simulink model "VVI_REPLACEMENT"  (R2022b)
settings: Solver=FixedStepAuto  StartTime=0.0  StopTime=100  FixedStep=1e-3  RelTol=1e-3  EnableMultiTasking=on
undefined symbols (not defined in the file): D1, D10, D12, D13, D2, D3, D5, D9, PTA1, PTA2, PTB9, PTC17, PTC4, PTD0, PTD1, PTD3
libraries: frdmk64flib x8
settings Model: ExtModeTrigDuration=5  Creator=aldenluscher  LastModifiedBy=aldenluscher
settings OptimizationCC: EnhancedBackFolding=on  PassReuseOutputArgsAs=Individual arguments  ZeroExternalMemoryAtStartup=off  ZeroInternalMemoryAtStartup=off  MaxStackSize=64  OptimizeBlockOrder=speed  DifferentSizesBufferReuse=on  OptimizationCustomize=off  EfficientTunableParamExpr=on
settings DebuggingCC: ParameterTunabilityLossMsg=error
settings HardwareCC: ProdBitPerPointer=32  ProdBitPerSizeT=32  ProdBitPerPtrDiffT=32  ProdLargestAtomicInteger=Long  ProdLargestAtomicFloat=Double  ProdWordSize=32  ProdHWDeviceType=ARM Compatible->ARM Cortex
settings SFSimCC: MATLABDynamicMemAlloc=off
settings RTWCC: Description=Embedded Coder  SystemTargetFile=ert.tlc  HardwareBoard=NXP FRDM-K64F  TLCOptions="-aInlineSetEventsForThisBaseRateFcn=TLC_FALSE -aSuppressMultiTaskScheduler=TLC_FALSE  -aRateBasedStepFcn=0"  TemplateMakefile=ert_default_tmf  Toolchain=GNU Tools for ARM Embedded Processors
settings CodeAppCC: ForceParamTrailComments=on  IgnoreCustomStorageClasses=off  OperatorAnnotations=on  SimulinkDataObjDesc=on  SFDataObjDesc=on  InsertBlockDesc=on
settings ERTTargetCC: ExtModeTransport=4  ExtModeMexFile=sendToCommService

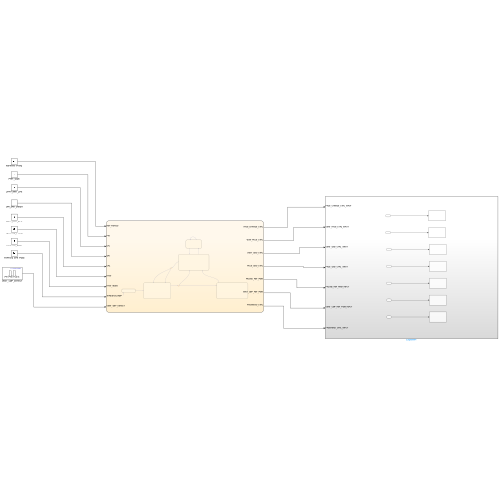
[thumbnail: Simulink's stored preview of the top-level diagram]
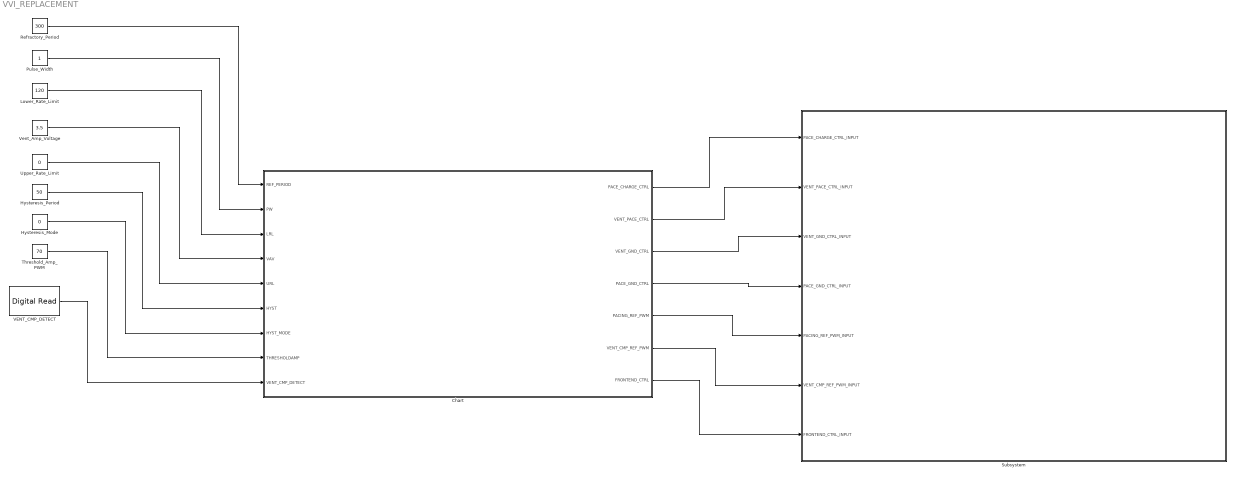
== system VVI_REPLACEMENT ==
  Chart : Stateflow chart  TreatAsAtomicUnit=on
      settings: PortSchema="{\"entries\":[{\"content\":{\"sides\":[{\"content\":{\"connectorIds\":[\"In1\",\"In2\",\"In3\",\"In4\",\"In5\",\"In7\",\"In6\",\"In9\",\"In8\"]},\"type\":\"ConnectorPlacement.EquallySpacedRectSide\",\"uuid\":\"2ae54867-0d42-4dc9-a711-c3558df1a1e5\"},{\"content\":{\"connectorIds\":[\"Out1\",\"Out2\",\"Out3\",\"Out4\",\"Out5\",\"Out6\",\"Out7\"],\"side\":\"RIGHT\"},\"type\":\"ConnectorPlacement.EquallySpacedRectSide\",\"uuid\":\"0827b622-949a-4894-bfc3-fcfa9f1c5c6f\"},{\"content\":{\"connectorIds\":[],\"side\":\"TOP\"},\"type\":\"ConnectorPlacement.EquallySpacedRectSide\",\"uuid\":\"b2dc8d34-414d-4327-a079-fe4380aaf0f4\"}]},\"type\":\"ConnectorPlacement.EquallySpacedConnector\",\"uuid\":\"8b20b6f2-40a5-4126-b6c0-e8236ebafa56\"}],\"packageUris\":[\"http://schema.mathworks.com/mf0/Connector/R2020b\"],\"version\":\"1.0\"}"
  Hysteresis_Mode : Constant  Value=0
  Hysteresis_Period : Constant  Value=50
  Lower_Rate_Limit : Constant  Value=120
  Pulse_Width : Constant
  Refractory_Period : Constant  Value=300
  Subsystem : Subsystem
  Threshold_Amp_PWM : Constant  Value=70
  Upper_Rate_Limit : Constant  Value=0
  VENT_CMP_DETECT : frdmk64flib/Digital Read  Whichpin=PTC17 (D1)  SampleTime=-1
  Vent_Amp_Voltage : Constant  Value=3.5
  wires:
  VENT_CMP_DETECT/1 -> Chart/8(VENT_CMP_DETECT)
  Threshold_Amp_PWM/1 -> Chart/9(THRESHOLDAMP)
  Chart/3(VENT_GND_CTRL) -> Subsystem/3(VENT_GND_CTRL_INPUT)
  Refractory_Period/1 -> Chart/1(REF_PERIOD)
  Vent_Amp_Voltage/1 -> Chart/4(VAV)
  Upper_Rate_Limit/1 -> Chart/5(URL)
  Chart/5(PACING_REF_PWM) -> Subsystem/5(PACING_REF_PWM_INPUT)
  Chart/6(VENT_CMP_REF_PWM) -> Subsystem/6(VENT_CMP_REF_PWM_INPUT)
  Hysteresis_Period/1 -> Chart/7(HYST)
  Hysteresis_Mode/1 -> Chart/6(HYST_MODE)
  Chart/2(VENT_PACE_CTRL) -> Subsystem/2(VENT_PACE_CTRL_INPUT)
  Chart/1(PACE_CHARGE_CTRL) -> Subsystem/1(PACE_CHARGE_CTRL_INPUT)
  Lower_Rate_Limit/1 -> Chart/3(LRL)
  Chart/7(FRONTEND_CTRL) -> Subsystem/7(FRONTEND_CTRL_INPUT)
  Pulse_Width/1 -> Chart/2(PW)
  Chart/4(PACE_GND_CTRL) -> Subsystem/4(PACE_GND_CTRL_INPUT)

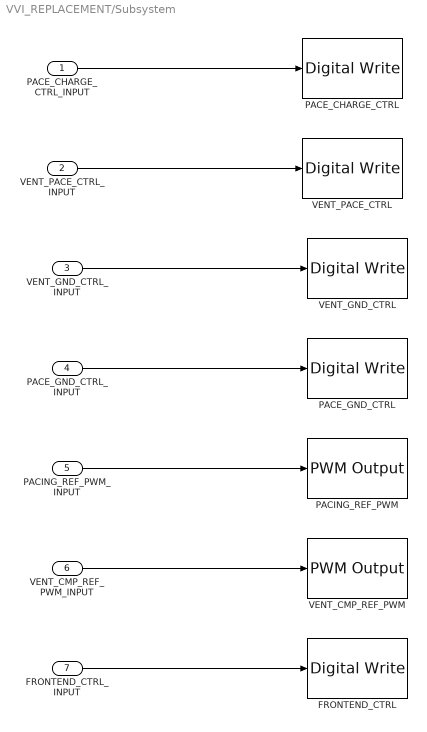
== system VVI_REPLACEMENT/Subsystem ==
  PACE_CHARGE_CTRL_INPUT : Inport
  VENT_PACE_CTRL_INPUT : Inport  Port=2
  VENT_GND_CTRL_INPUT : Inport  Port=3
  PACE_GND_CTRL_INPUT : Inport  Port=4
  PACING_REF_PWM_INPUT : Inport  Port=5
  VENT_CMP_REF_PWM_INPUT : Inport  Port=6
  FRONTEND_CTRL_INPUT : Inport  Port=7
  FRONTEND_CTRL : frdmk64flib/Digital Write  Whichpin=PTD1 (D13)
  PACE_CHARGE_CTRL : frdmk64flib/Digital Write  Whichpin=PTB9 (D2)
  PACE_GND_CTRL : frdmk64flib/Digital Write  Whichpin=PTD0 (D10)
  PACING_REF_PWM : frdmk64flib/PWM Output  Whichpin=PTA2 (D5)  InitialFrequency=2000  InitialDutyCycle=0
  VENT_CMP_REF_PWM : frdmk64flib/PWM Output  Whichpin=PTA1 (D3)  InitialFrequency=2000  InitialDutyCycle=0
  VENT_GND_CTRL : frdmk64flib/Digital Write  Whichpin=PTD3 (D12)
  VENT_PACE_CTRL : frdmk64flib/Digital Write  Whichpin=PTC4 (D9)
  wires:
  VENT_PACE_CTRL_INPUT/1 -> VENT_PACE_CTRL/1
  PACE_GND_CTRL_INPUT/1 -> PACE_GND_CTRL/1
  PACE_CHARGE_CTRL_INPUT/1 -> PACE_CHARGE_CTRL/1
  PACING_REF_PWM_INPUT/1 -> PACING_REF_PWM/1
  VENT_GND_CTRL_INPUT/1 -> VENT_GND_CTRL/1
  VENT_CMP_REF_PWM_INPUT/1 -> VENT_CMP_REF_PWM/1
  FRONTEND_CTRL_INPUT/1 -> FRONTEND_CTRL/1

== stateflow chart VVI_REPLACEMENT/Chart ==
  state Timing_Natural_PW_in_msec_
    NAT_PW=NAT_PW+1;
  state Refractory_Period_
    PACE_CHARGE_CTRL = 1;
    PACE_GND_CTRL = 1;
    VENT_GND_CTRL = 1;
    VENT_PACE_CTRL = 0;
  state Charging_
    PACING_REF_PWM = 100*(VAV/5);
    PACING_PERIOD = (60000/LRL);
    HYST_PERIOD = (60000/HYST);
    PACE_CHARGE_CTRL = 1;
    PACE_GND_CTRL = 1;
    VENT_GND_CTRL = 1;
    VENT_PACE_CTRL = 0;
    VENT_CMP_REF_PWM = THRESHOLDAMP;
    FRONTEND_CTRL = 1;
    NAT_PW = 0;
    TOTAL_NAT_PW = 0;
    PACE_PW = 0;
  state Pacing_
    PACE_CHARGE_CTRL = 0;
    PACE_GND_CTRL = 1;
    VENT_GND_CTRL = 0;
    VENT_PACE_CTRL = 1;
  state Setting_Initial_Period_
    PERIOD = (60000/LRL);
  Timing_Natural_PW_in_msec_ -> Timing_Natural_PW_in_msec_ [order 2] : after(1,msec)
  Timing_Natural_PW_in_msec_ -> Refractory_Period_ [order 1] : [VENT_CMP_DETECT==0]{TOTAL_NAT_PW = TOTAL_NAT_PW + NAT_PW}
  Refractory_Period_ -> Timing_Natural_PW_in_msec_ [order 1] : [VENT_CMP_DETECT==1]
  Refractory_Period_ -> (junction 15) [order 2] : after(REF_PERIOD-PACE_PW-TOTAL_NAT_PW,msec)
  (junction 15) -> Charging_ [order 1] : [HYST_MODE == 1]{PERIOD = HYST_PERIOD}
  (junction 15) -> Charging_ [order 2] : [HYST_MODE == 0]{PERIOD = PACING_PERIOD}
  (junction 4) -> Refractory_Period_ [order 2] : [VENT_CMP_DETECT == 1]
  Pacing_ -> Refractory_Period_ : after(PW,msec){PACE_PW = PW}
  Charging_ -> (junction 4)
  (junction 4) -> Pacing_ [order 1] : after(PERIOD-PW-REF_PERIOD,msec)[VENT_CMP_DETECT == 0]
  Setting_Initial_Period_ -> Charging_
  (default) -> Setting_Initial_Period_
  data: REF_PERIOD input; PW input; LRL input; VAV input; URL input; HYST_MODE input; HYST input; PACE_CHARGE_CTRL output; VENT_PACE_CTRL output; VENT_GND_CTRL output; PACE_GND_CTRL output; PACING_REF_PWM output; VENT_CMP_DETECT input; VENT_CMP_REF_PWM output; PACING_PERIOD local; PERIOD local; HYST_PERIOD local; THRESHOLDAMP input; FRONTEND_CTRL output; NAT_PW local; TOTAL_NAT_PW local; PACE_PW local
